simulink subsystem "nlinear"  (R2023a)
settings: Solver=VariableStepAuto  StartTime=0.0  StopTime=10.0  RelTol=1e-3
undefined symbols (not defined in the file): v_ic, x_ic
settings Model: Creator=pinki  LastModifiedBy=pinki

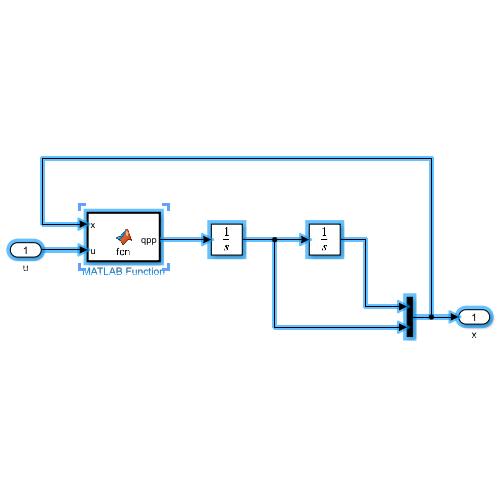
[thumbnail: Simulink's stored preview of the top-level diagram]
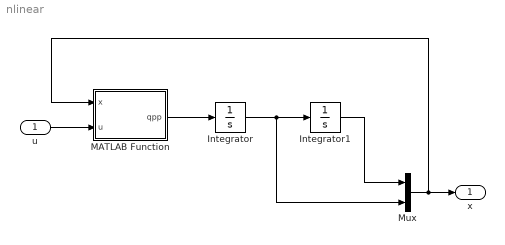
== system nlinear ==
  u : Inport
  Integrator : Integrator  InitialCondition=v_ic
  Integrator1 : Integrator  InitialCondition=x_ic
  MATLAB Function : MATLAB Function  TreatAsAtomicUnit=on
  Mux : Mux  Inputs=2
  x : Outport
  wires:
  Integrator/1 -> Mux/2, Integrator1/1
  Mux/1 -> MATLAB Function/1(x), x/1
  u/1 -> MATLAB Function/2(u)
  Integrator1/1 -> Mux/1
  MATLAB Function/1(qpp) -> Integrator/1

== matlab function nlinear/MATLAB Function ==
  data: x input; u input; qpp output
function qpp = fcn(x,u)

M = function_M(x(4));
V = function_V(x(6),x(4),x(8),x(5),x(7));
G = function_G(x(2),x(4));
P = function_P();

qpp = M^-1*(-V-G+P*u);
